simulink model "SIMrun_H_LIP"  (R2024b)
settings: Solver=FixedStepDiscrete  StartTime=0.0  StopTime=50  FixedStep=Ts+Td  RelTol=1e-3
values from neighbouring files (symbols this model uses):
  K = [1, Td + (1/ld)*coth(ld*Ts)]    [H_LIP_main_analytical.m]    (also in H_LIP_main_ode45_solver.m)
  ld = sqrt(g/z0)    [H_LIP_main_analytical.m]    (also in H_LIP_main_ode45_solver.m)
  Td = 0.1    [H_LIP_main_analytical.m]    (also in H_LIP_main_ode45_solver.m)
  Ts = 0.2    [H_LIP_main_analytical.m]    (also in H_LIP_main_ode45_solver.m; LIP_main.m = 0.35)
  ud = xd(2)*(Ts + Td)    [H_LIP_main_analytical.m]    (also in H_LIP_main_ode45_solver.m)
  vi = 0.5    [H_LIP_main_analytical.m]
  xd = [-0.1;1]    [H_LIP_main_analytical.m]    (also in H_LIP_main_ode45_solver.m; LIP_main.m = 0.1)
  xi = -0.05    [H_LIP_main_analytical.m]    (also in H_LIP_main_ode45_solver.m = [-0.05;0.5])
settings Model: Creator=FurusTM  LastModifiedBy=FurusTM

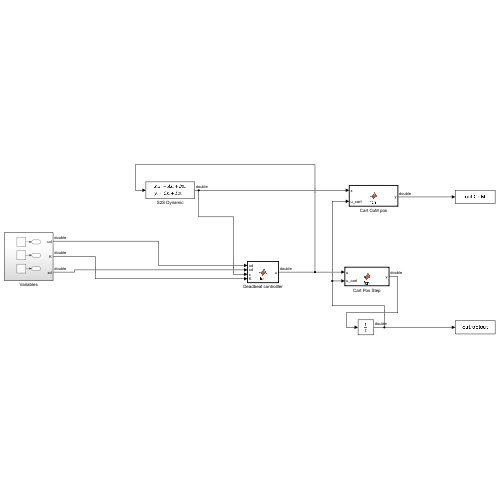
[thumbnail: Simulink's stored preview of the top-level diagram]
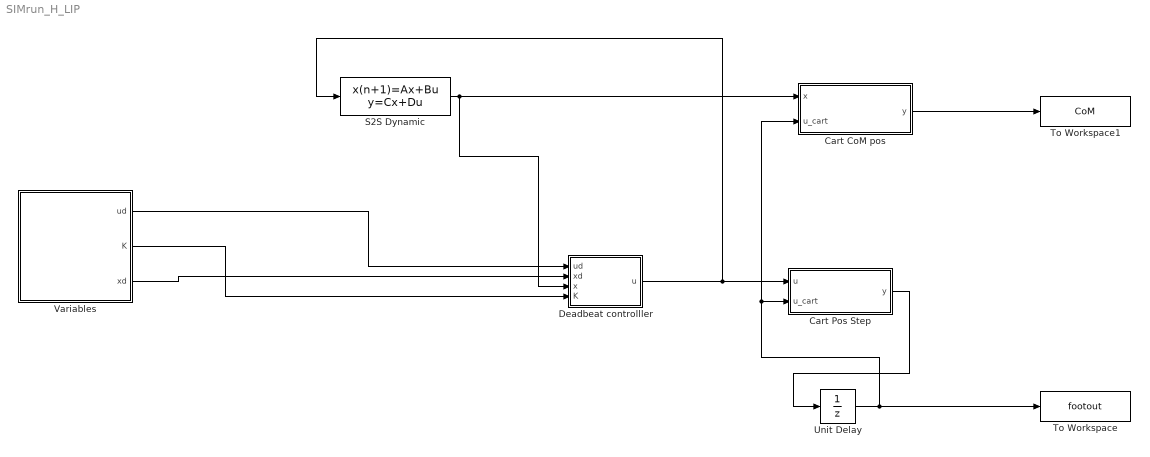
== system SIMrun_H_LIP ==
  Cart CoM pos : MATLAB Function  TreatAsAtomicUnit=on
  Cart Pos Step : MATLAB Function  TreatAsAtomicUnit=on
  Deadbeat controlller : MATLAB Function  TreatAsAtomicUnit=on
  S2S Dynamic : DiscreteStateSpace  A=[cosh(ld*Ts) + ld*Td*sinh(ld*Ts), (1/ld)*sinh(ld*Ts) + Td*cosh(ld*Ts); ld*sinh(ld*Ts), cosh(ld*Ts)]  B=[-1;0]  C=eye(2)  D=zeros(2,1)  InitialCondition=[xi;vi]  SampleTime=-1
  To Workspace : ToWorkspace  VariableName=footout  SaveFormat=Timeseries  SampleTime=-1
  To Workspace1 : ToWorkspace  VariableName=CoM  SaveFormat=Timeseries  SampleTime=-1
  Unit Delay : UnitDelay  SampleTime=-1  HasFrameUpgradeWarning=on
  Variables : Subsystem
  wires:
  Deadbeat controlller/1(u) -> Cart Pos Step/1(u), S2S Dynamic/1
  Variables/1(ud) -> Deadbeat controlller/1(ud)
  Variables/2(K) -> Deadbeat controlller/4(K)
  Variables/3(xd) -> Deadbeat controlller/2(xd)
  Cart Pos Step/1(y) -> Unit Delay/1
  Unit Delay/1 -> To Workspace/1, Cart CoM pos/2(u_cart), Cart Pos Step/2(u_cart)
  Cart CoM pos/1(y) -> To Workspace1/1
  S2S Dynamic/1 -> Deadbeat controlller/3(x), Cart CoM pos/1(x)

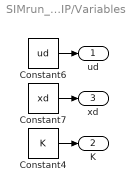
== system SIMrun_H_LIP/Variables ==
  Constant4 : Constant  Value=K
  Constant6 : Constant  Value=ud
  Constant7 : Constant  Value=xd
  ud : Outport
  K : Outport  Port=2
  xd : Outport  Port=3
  wires:
  Constant4/1 -> K/1
  Constant6/1 -> ud/1
  Constant7/1 -> xd/1

== matlab function SIMrun_H_LIP/Cart Pos Step ==
  data: u input; y output; u_cart input
function y = fcn(u,u_cart)

y = u + u_cart;

== matlab function SIMrun_H_LIP/Deadbeat controlller ==
  data: ud input; u output; xd input; x input; K input
function u = fcn(ud,xd,x,K)

% Force shapes (Simulink often sends x as width-2 vector)
x  = x(:);          % 2x1
xd = xd(:);         % 2x1
K  = reshape(K,1,2);% 1x2

a = K * (x - xd);
u = ud + a;

== matlab function SIMrun_H_LIP/Cart CoM pos ==
  data: x input; y output; u_cart input
function y = fcn(x,u_cart)

y = x(1) + u_cart;
